simulink model "DC_motor"  (R2017a)
settings: Solver=VariableStepAuto  StartTime=0.0  StopTime=10  RelTol=1e-5
undefined symbols (not defined in the file or in its folder): b, J, Kphi, L, R, sigbuilder_block
libraries: simulink x1
settings Model: Creator=samir  LastModifiedBy=samir

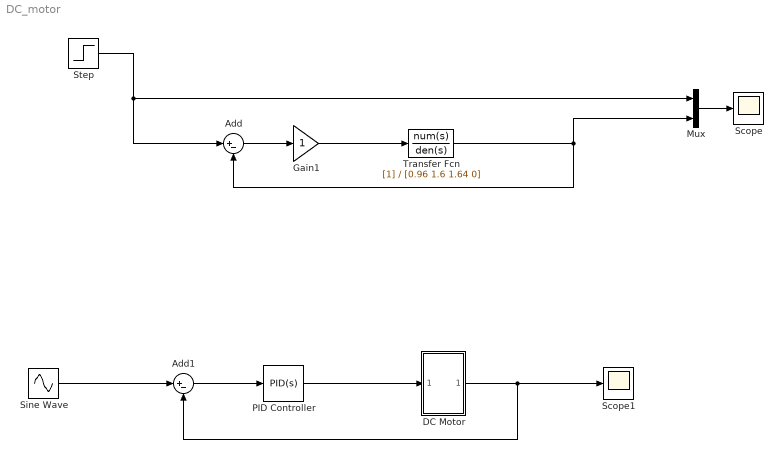
== system DC_motor ==
  Add : Sum  Inputs=|+-
  Add1 : Sum  Inputs=|+-
  DC Motor : Subsystem
  Gain1 : Gain
  Mux : Mux  Inputs=2
  PID Controller : simulink/Continuous/PID Controller  Controller=PID  TimeDomain=Continuous-time  SampleTime=-1  IntegratorMethod=Forward Euler  FilterMethod=Forward Euler  Form=Parallel  UseFilter=on  ControllerParametersSource=internal  P=1  I=0.6  D=0  N=100  InitialConditionSource=internal  InitialConditionForIntegrator=0  InitialConditionForFilter=0  ExternalReset=none  LimitOutput=off  UpperSaturationLimit=inf  LowerSaturationLimit=-inf  LinearizeAsGain=on  AntiWindupMode=none  Kb=1  TrackingMode=off  Kt=1  PParamMin=[]  PParamMax=[]  IParamMin=[]  IParamMax=[]  DParamMin=[]  DParamMax=[]  NParamMin=[]  NParamMax=[]  KbParamMin=[]  KbParamMax=[]  KtParamMin=[]  KtParamMax=[]  POutMin=[]  POutMax=[]  IOutMin=[]  IOutMax=[]  DOutMin=[]  DOutMax=[]  NOutMin=[]  NOutMax=[]  KbOutMin=[]  KbOutMax=[]  KtOutMin=[]  KtOutMax=[]  IntegratorOutMin=[]  IntegratorOutMax=[]  FilterOutMin=[]  FilterOutMax=[]  SumOutMin=[]  SumOutMax=[]  SumI1OutMin=[]  SumI1OutMax=[]  SumI2OutMin=[]  SumI2OutMax=[]  SumI3OutMin=[]  SumI3OutMax=[]  SumDOutMin=[]  SumDOutMax=[]  SaturationOutMin=[]  SaturationOutMax=[]  IntegratorContinuousStateAttributes=''  IntegratorStateMustResolveToSignalObject=off  IntegratorRTWStateStorageClass=Auto  FilterContinuousStateAttributes=''  FilterStateMustResolveToSignalObject=off  FilterRTWStateStorageClass=Auto  DifferentiatorICPrevScaledInput=0  DifferentiatorOutMin=[]  DifferentiatorOutMax=[]  InitialConditionSetting=State (most efficient)
  Scope : Scope
  Scope1 : Scope
  Sine Wave : Sin  Frequency=5*2*pi  SampleTime=0
  Step : Step  Time=0  SampleTime=0
  Transfer Fcn : TransferFcn  Denominator=[0.96 1.6 1.64 0]
  wires:
  Add/1 -> Gain1/1
  Mux/1 -> Scope/1
  Gain1/1 -> Transfer Fcn/1
  Step/1 -> Add/1, Mux/1
  Transfer Fcn/1 -> Add/2, Mux/2
  Sine Wave/1 -> Add1/1
  Add1/1 -> PID Controller/1
  DC Motor/1(Out1) -> Add1/2, Scope1/1
  PID Controller/1 -> DC Motor/1(In1)

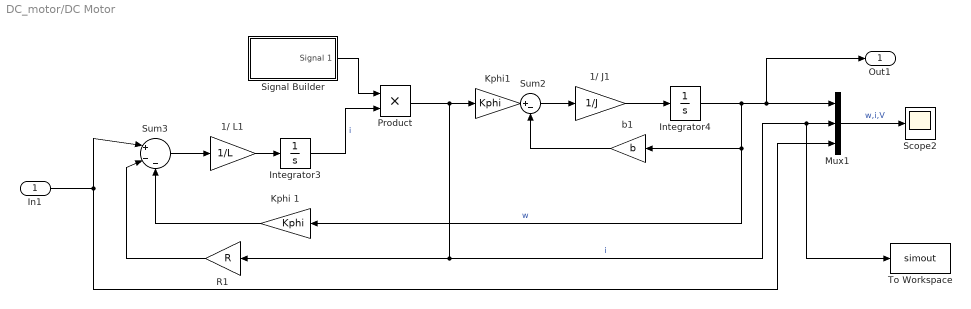
== system DC_motor/DC Motor ==
  In1 : Inport
  1/ J1 : Gain  Gain=1/J
  1/ L1 : Gain  Gain=1/L
  Integrator3 : Integrator
  Integrator4 : Integrator
  Kphi 1 : Gain  Gain=Kphi
  Kphi1 : Gain  Gain=Kphi
  Mux1 : Mux  Inputs=3
  Product : Product
  R1 : Gain  Gain=R
  Scope2 : Scope
  Signal Builder : Subsystem  Tag=STV Subsys  LoadFcn=sigbuilder_block('load');  StartFcn=sigbuilder_block('start');  StopFcn=sigbuilder_block('stop');  ClipboardFcn=sigbuilder_block('clipboard');  mask(Sigbuilder block){tuvar=[0:10]}
      mask help: Simulink:masks:SigbuilderBlock_MD
      mask init:
      | if ~strcmp(get_param(bdroot(gcbh),'SimulationStatus'),'stopped') tuvar = sigbuilder_block('maskInit'); end
      settings: CopyFcn=sigbuilder_block('copy');  DeleteFcn=sigbuilder_block('delete');  ModelCloseFcn=sigbuilder_block('modelClose');  PreSaveFcn=sigbuilder_block('preSave');  PauseFcn=sigbuilder_block('pause');  ContinueFcn=sigbuilder_block('continue');  NameChangeFcn=sigbuilder_block('namechange');  OpenFcn=sigbuilder_block('open',[404 117.5 550.5 362.5 ]);  CloseFcn=sigbuilder_block('close');
      mask Display: plot(0, 0, 100, 100,[2, 2, 32, 32, 2], [68, 8, 8, 68, 68],[32, 2], [38, 38], [32, 19, 2],[53, 60, 44], [32, 17, 17, 2],[16, 16, 31, 31]);txt = getActiveGroup(gcbh);text(2, 100, txt,'verticalAlignment', 'top');
  Sum2 : Sum  Inputs=|+-
  Sum3 : Sum  Inputs=|+--
  To Workspace : ToWorkspace  VariableName=simout  SampleTime=-1
  b1 : Gain  Gain=b
  Out1 : Outport
  wires:
  Product/1 -> R1/1, To Workspace/1, Mux1/2, Kphi1/1  "i"
  Kphi1/1 -> Sum2/1
  1/ J1/1 -> Integrator4/1
  Mux1/1 -> Scope2/1  "w,i,V"
  In1/1 -> Sum3/1, Mux1/3
  1/ L1/1 -> Integrator3/1
  Sum3/1 -> 1/ L1/1
  Integrator4/1 -> b1/1, Kphi 1/1, Out1/1, Mux1/1  "w"
  Kphi 1/1 -> Sum3/3
  b1/1 -> Sum2/2
  R1/1 -> Sum3/2
  Sum2/1 -> 1/ J1/1
  Integrator3/1 -> Product/2  "i"
  Signal Builder/1(Signal 1) -> Product/1

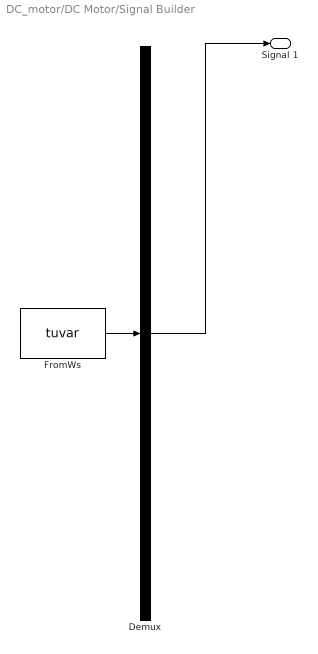
== system DC_motor/DC Motor/Signal Builder ==
  Demux : Demux  Tag=STV Demux  Outputs=1
  FromWs : FromWorkspace  Tag=STV FromWs  VariableName=tuvar  SampleTime=0
      SigBuilderData=|
      | common.afterFinalStr = 'Extrapolate'
      | common.sampleTime = 0
      | dataSet.timeRange = [0 10]
      | dataSet.name = 'Group 1'
      | sbobj.Groups.Name = 'Group 1'
      | sbobj.Groups.Signals.Name = 'Signal 1'
      | sbobj.Groups.Signals.XData = [0 2.3 2.3 2.48 2.48 4.98 4.98 5.18 5.18 10]
      | sbobj.Groups.Signals.YData = [0.995 0.995 0.6 0.6 0.995 0.995 0.19 0.19 0.995 0.995]
  Signal 1 : Outport  Tag=STV Outport
  wires:
  Demux/1 -> Signal 1/1
  FromWs/1 -> Demux/1
